simulink model "morus_uav_smc_DOB"  (R2016b)
settings: Solver=FixedStepAuto  StartTime=0.0  StopTime=15  FixedStep=0.001  MaxStep=0.001  RelTol=1e-5  EnableMultiTasking=on
values from neighbouring files (symbols this model uses):
  b_gm_f = F_n / (w_gm_n^2)    (= 0.000456410576724)    [morus_uav_params.m]
  b_gm_m = 0.01    [morus_uav_params.m]
  beta = deg2rad(0)    [morus_uav_params.m]
  cd = 0    [morus_uav_params.m]
  g = 9.81    [morus_uav_params.m]
  Iq = [Iq_xx 0 0; 0 Iq_yy 0; 0 0 Iq_zz]    [morus_uav_params.m]
  Iq_yy = 0.00528250    (= 0.0052825)    [morus_uav_params.m]
  kd_mp = 0.015    [morus_uav_params.m]
  kd_mv = 0.01    [morus_uav_params.m]
  kd_vz = 10    [morus_uav_params.m]
  kd_z = 1    [morus_uav_params.m]
  ki_mp = 0.25    [morus_uav_params.m]
  ki_mv = 06    (= 6)    [morus_uav_params.m]
  ki_vz = 20    [morus_uav_params.m]
  ki_z = 0    [morus_uav_params.m]
  Km = 1    [morus_uav_params.m]
  kp_mp = 25    [morus_uav_params.m]
  kp_mv = 0.6    [morus_uav_params.m]
  kp_vz = 75    [morus_uav_params.m]
  kp_z = 4    [morus_uav_params.m]
  l_rot = 0.265    [morus_uav_params.m]
  lm = 0.17    [morus_uav_params.m]
  m = 0.208    [morus_uav_params.m]
  M = mq + 4 * m    (= 2.915)    [morus_uav_params.m]
  mq = 2.083    [morus_uav_params.m]
  T_obz1 = 5    [morus_uav_params.m]
  T_obz2 = 5    [morus_uav_params.m]
  Tf1 = 0.12    [morus_uav_params.m]
  Tf2 = 0.12    [morus_uav_params.m]
  Tgm = 0.2    [morus_uav_params.m]
  Tr = 12.24268    [morus_uav_params.m]
  w_gm_0 = sqrt(M*g/4/b_gm_f)    [morus_uav_params.m]
  zeta = [1 -1 1 -1]    [morus_uav_params.m]
  zm = 0    [morus_uav_params.m]
libraries: aerolibutil x20, simulink x10, dspmtrx3 x5, aerolibtransform2 x4
(part 1 of 2)
settings Model: Creator=tomislav  LastModifiedBy=martinatomic
settings DataIOCC: LimitDataPoints=on  SaveFormat=Array
settings OptimizationCC: LifeSpan=inf
settings DebuggingCC: SFUnexpectedBacktrackingDiag=warning  SFNoUnconditionalDefaultTransitionDiag=warning  SFExecutionAtInitializationDiag=none
settings HardwareCC: ProdBitPerPointer=32  ProdBitPerSizeT=32  ProdBitPerPtrDiffT=32  ProdLargestAtomicFloat=None  ProdIntDivRoundTo=Undefined  ProdEndianess=Unspecified  ProdWordSize=32  ProdHWDeviceType=32-bit Generic
settings ModelReferenceCC: PropagateSignalLabelsOutOfModel=off
settings GRTTargetCC: TargetLangStandard=C89/C90 (ANSI)  GeneratePreprocessorConditionals=Disable all
settings ConfigComp: CovMetricSettings=dw  CovHtmlReporting=on  CovSaveCumulativeToWorkspaceVar=on  CovSaveSingleToWorkspaceVar=on  CovExternalEMLEnable=off

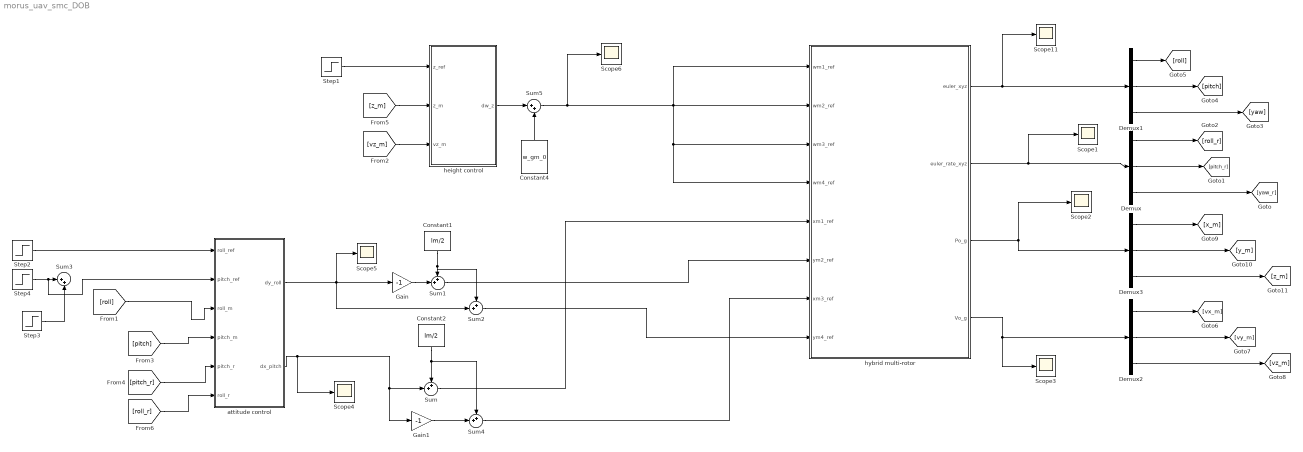
== system morus_uav_smc_DOB ==
  Constant1 : Constant  Value=lm/2
  Constant2 : Constant  Value=lm/2
  Constant4 : Constant  Value=w_gm_0
  Demux{,1..3} (4 alike) : Demux  Outputs=3
  Gain : Gain  Gain=-1
  Gain1 : Gain  Gain=-1
  Scope{1..6,11} (7 alike) : Scope
  Step1 : Step  Time=0  SampleTime=0
  Step2 : Step  Time=5  After=-0.1  SampleTime=0
  Step3 : Step  Time=9  After=0.1  SampleTime=0
  Step4 : Step  Time=5  After=0.1  SampleTime=0
  Sum{,1..2,4} (4 alike) : Sum  Inputs=++|
  Sum3 : Sum  Inputs=|++
  Sum5 : Sum  Inputs=|++
  attitude control : Subsystem
  height control : Subsystem
  hybrid multi-rotor : Subsystem
  wires:
  Sum2/1 -> hybrid multi-rotor/8(ym4_ref)
  hybrid multi-rotor/1(euler_xyz) -> Demux1/1, Scope11/1
  hybrid multi-rotor/2(euler_rate_xyz) -> Demux/1, Scope1/1
  Demux/2 -> [pitch_r]
  Demux1/2 -> [pitch]
  Sum5/1 -> Scope6/1, hybrid multi-rotor/1(wm1_ref), hybrid multi-rotor/4(wm4_ref), hybrid multi-rotor/3(wm3_ref), hybrid multi-rotor/2(wm2_ref)
  height control/1(dw_z) -> Sum5/1
  Constant4/1 -> Sum5/2
  hybrid multi-rotor/4(Vo_g) -> Demux2/1, Scope3/1
  Demux2/2 -> [vy_m]
  Demux2/3 -> [vz_m]
  Demux2/1 -> [vx_m]
  hybrid multi-rotor/3(Po_g) -> Demux3/1, Scope2/1
  Demux3/2 -> [y_m]
  Demux3/3 -> [z_m]
  Demux3/1 -> [x_m]
  [vz_m] -> height control/3(vz_m)
  [z_m] -> height control/2(z_m)
  Step1/1 -> height control/1(z_ref)
  Constant1/1 -> Sum2/1, Sum1/1
  Gain/1 -> Sum1/2
  Constant2/1 -> Sum/1, Sum4/1
  Gain1/1 -> Sum4/2
  Sum/1 -> hybrid multi-rotor/5(xm1_ref)
  Sum1/1 -> hybrid multi-rotor/6(ym2_ref)
  Sum4/1 -> hybrid multi-rotor/7(xm3_ref)
  Step2/1 -> attitude control/1(roll_ref)
  attitude control/2(dx_pitch) -> Sum/2, Gain1/1, Scope4/1
  [pitch] -> attitude control/4(pitch_m)
  [roll] -> attitude control/3(roll_m)
  attitude control/1(dy_roll) -> Scope5/1, Sum2/2, Gain/1
  Demux/1 -> [roll_r]
  Demux/3 -> [yaw_r]
  Demux1/1 -> [roll]
  Demux1/3 -> [yaw]
  [pitch_r] -> attitude control/5(pitch_r)
  [roll_r] -> attitude control/6(roll_r)
  Step4/1 -> attitude control/2(pitch_ref), Sum3/1
  Step3/1 -> Sum3/2

== system morus_uav_smc_DOB/attitude control ==
  roll_ref : Inport
  pitch_ref : Inport  Port=2
  roll_m : Inport  Port=3
  pitch_m : Inport  Port=4
  pitch_r : Inport  Port=5
  roll_r : Inport  Port=6
  pitch control : Subsystem
  roll control : Subsystem
  dy_roll : Outport
  dx_pitch : Outport  Port=2
  wires:
  pitch_ref/1 -> pitch control/1(pitch_ref)
  pitch control/1(dx_pitch) -> dx_pitch/1
  pitch_m/1 -> pitch control/2(pitch_m)
  roll control/1(dy_roll) -> dy_roll/1
  roll_m/1 -> roll control/2(roll_m)
  roll_ref/1 -> roll control/1(roll_ref)
  pitch_r/1 -> pitch control/3(pitch_r)
  roll_r/1 -> roll control/3(roll_r)

== system morus_uav_smc_DOB/height control ==
  z_ref : Inport
  z_m : Inport  Port=2
  vz_m : Inport  Port=3
  Mux : Mux  Inputs=2
  Mux1 : Mux  Inputs=2
  PID Controller : simulink/Continuous/PID Controller  Controller=PID  TimeDomain=Continuous-time  SampleTime=-1  IntegratorMethod=Forward Euler  FilterMethod=Forward Euler  Form=Parallel  UseFilter=on  ControllerParametersSource=internal  P=kp_vz  I=ki_vz  D=kd_vz  N=100  InitialConditionSource=internal  InitialConditionForIntegrator=0  InitialConditionForFilter=0  ExternalReset=none  LimitOutput=on  UpperSaturationLimit=400  LowerSaturationLimit=-400  LinearizeAsGain=on  AntiWindupMode=clamping  Kb=1  TrackingMode=off  Kt=1  PParamMin=[]  PParamMax=[]  IParamMin=[]  IParamMax=[]  DParamMin=[]  DParamMax=[]  NParamMin=[]  NParamMax=[]  KbParamMin=[]  KbParamMax=[]  KtParamMin=[]  KtParamMax=[]  POutMin=[]  POutMax=[]  IOutMin=[]  IOutMax=[]  DOutMin=[]  DOutMax=[]  NOutMin=[]  NOutMax=[]  KbOutMin=[]  KbOutMax=[]  KtOutMin=[]  KtOutMax=[]  IntegratorOutMin=[]  IntegratorOutMax=[]  FilterOutMin=[]  FilterOutMax=[]  SumOutMin=[]  SumOutMax=[]  SumI1OutMin=[]  SumI1OutMax=[]  SumI2OutMin=[]  SumI2OutMax=[]  SumI3OutMin=[]  SumI3OutMax=[]  SumDOutMin=[]  SumDOutMax=[]  SaturationOutMin=[]  SaturationOutMax=[]  IntegratorContinuousStateAttributes=''  IntegratorStateMustResolveToSignalObject=off  IntegratorRTWStateStorageClass=Auto  FilterContinuousStateAttributes=''  FilterStateMustResolveToSignalObject=off  FilterRTWStateStorageClass=Auto  DifferentiatorICPrevScaledInput=0  DifferentiatorOutMin=[]  DifferentiatorOutMax=[]
  PID Controller1 : simulink/Continuous/PID Controller  Controller=PID  TimeDomain=Continuous-time  SampleTime=-1  IntegratorMethod=Forward Euler  FilterMethod=Forward Euler  Form=Parallel  UseFilter=on  ControllerParametersSource=internal  P=kp_z  I=ki_z  D=kd_z  N=100  InitialConditionSource=internal  InitialConditionForIntegrator=0  InitialConditionForFilter=0  ExternalReset=none  LimitOutput=on  UpperSaturationLimit=5  LowerSaturationLimit=-5  LinearizeAsGain=on  AntiWindupMode=clamping  Kb=1  TrackingMode=off  Kt=1  PParamMin=[]  PParamMax=[]  IParamMin=[]  IParamMax=[]  DParamMin=[]  DParamMax=[]  NParamMin=[]  NParamMax=[]  KbParamMin=[]  KbParamMax=[]  KtParamMin=[]  KtParamMax=[]  POutMin=[]  POutMax=[]  IOutMin=[]  IOutMax=[]  DOutMin=[]  DOutMax=[]  NOutMin=[]  NOutMax=[]  KbOutMin=[]  KbOutMax=[]  KtOutMin=[]  KtOutMax=[]  IntegratorOutMin=[]  IntegratorOutMax=[]  FilterOutMin=[]  FilterOutMax=[]  SumOutMin=[]  SumOutMax=[]  SumI1OutMin=[]  SumI1OutMax=[]  SumI2OutMin=[]  SumI2OutMax=[]  SumI3OutMin=[]  SumI3OutMax=[]  SumDOutMin=[]  SumDOutMax=[]  SaturationOutMin=[]  SaturationOutMax=[]  IntegratorContinuousStateAttributes=''  IntegratorStateMustResolveToSignalObject=off  IntegratorRTWStateStorageClass=Auto  FilterContinuousStateAttributes=''  FilterStateMustResolveToSignalObject=off  FilterRTWStateStorageClass=Auto  DifferentiatorICPrevScaledInput=0  DifferentiatorOutMin=[]  DifferentiatorOutMax=[]
  Scope1 : Scope
  Scope4 : Scope
  Scope6 : Scope
  Sum : Sum  Inputs=|+-
  Sum1 : Sum  Inputs=|+-
  dw_z : Outport
  wires:
  z_m/1 -> Sum1/2, Mux1/2
  Mux1/1 -> Scope6/1
  z_ref/1 -> Sum1/1, Mux1/1
  Sum/1 -> PID Controller/1
  Sum1/1 -> PID Controller1/1
  Mux/1 -> Scope4/1
  vz_m/1 -> Sum/2, Mux/2
  PID Controller1/1 -> Sum/1, Mux/1
  PID Controller/1 -> Scope1/1, dw_z/1

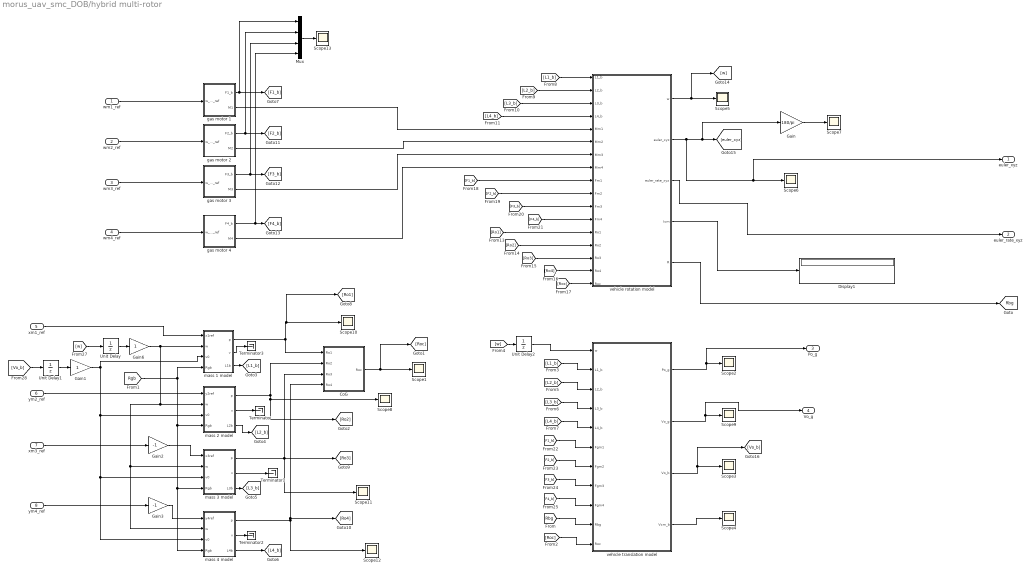
== system morus_uav_smc_DOB/hybrid multi-rotor ==
  wm1_ref : Inport
  wm2_ref : Inport  Port=2
  wm3_ref : Inport  Port=3
  wm4_ref : Inport  Port=4
  xm1_ref : Inport  Port=5
  ym2_ref : Inport  Port=6
  xm3_ref : Inport  Port=7
  ym4_ref : Inport  Port=8
  CoG : Subsystem
  Display1 : Display
  Gain : Gain  Gain=180/pi
  Gain1 : Gain
  Gain2 : Gain  Gain=-1
  Gain3 : Gain  Gain=-1
  Gain6 : Gain
  Mux : Mux
  Scope{1..13} (13 alike) : Scope
  Terminator{,1..3} (4 alike) : Terminator
  Unit Delay : UnitDelay  SampleTime=-1
  Unit Delay1 : UnitDelay  SampleTime=-1
  Unit Delay2 : UnitDelay  SampleTime=-1
  gas motor 1 : Subsystem
  gas motor 2 : Subsystem
  gas motor 3 : Subsystem
  gas motor 4 : Subsystem
  mass 1 model : Subsystem
  mass 2 model : Subsystem
  mass 3 model : Subsystem
  mass 4 model : Subsystem
  vehicle rotation model : Subsystem
  vehicle translation model : Subsystem
  euler_xyz : Outport
  euler_rate_xyz : Outport  Port=2
  Po_g : Outport  Port=3
  Vo_g : Outport  Port=4
  tag scope: Rbg=global
  wires:
  vehicle rotation model/3(euler_rate_xyz) -> euler_rate_xyz/1
  [Rbg] -> vehicle translation model/10(Rbg)
  mass 2 model/1(p) -> Scope8/1, [Ro2], CoG/2(Ro2)
  mass 3 model/1(p) -> CoG/3(Ro3), Scope11/1, [Ro3]
  mass 4 model/1(p) -> [Ro4], CoG/4(Ro4), Scope12/1
  [Roc] -> vehicle translation model/11(Roc)
  vehicle translation model/2(Vo_g) -> Vo_g/1, Scope9/1
  [Roc] -> vehicle rotation model/17(Roc)
  Gain2/1 -> mass 3 model/1(x3ref)
  [L1_b] -> vehicle rotation model/1(L1_b)
  mass 3 model/3(L3b) -> [L3_b]
  [L4_b] -> vehicle translation model/5(L4_b)
  [L2_b] -> vehicle translation model/3(L2_b)
  [Ro3] -> vehicle rotation model/15(Ro3)
  vehicle translation model/1(Po_g) -> Po_g/1, Scope2/1
  vehicle translation model/3(Vo_b) -> [Vo_b], Scope3/1
  mass 2 model/3(L2b) -> [L2_b]
  vehicle translation model/4(Vcm_b) -> Scope4/1
  xm1_ref/1 -> mass 1 model/1(x1ref)
  [Ro1] -> vehicle rotation model/13(Ro1)
  Gain3/1 -> mass 4 model/1(y4ref)
  [L3_b] -> vehicle rotation model/3(L3_b)
  [L3_b] -> vehicle translation model/4(L3_b)
  mass 1 model/3(L1b) -> [L1_b]
  [L2_b] -> vehicle rotation model/2(L2_b)
  [Ro4] -> vehicle rotation model/16(Ro4)
  [L1_b] -> vehicle translation model/2(L1_b)
  ym4_ref/1 -> Gain3/1
  [Ro2] -> vehicle rotation model/14(Ro2)
  vehicle rotation model/1(w) -> [w], Scope5/1
  vehicle rotation model/4(Icm) -> Display1/1
  ym2_ref/1 -> mass 2 model/1(y2ref)
  mass 4 model/3(L4b) -> [L4_b]
  xm3_ref/1 -> Gain2/1
  [F4_b] -> vehicle rotation model/12(Fm4)
  gas motor 2/1(F2_b) -> Mux/2, [F2_b]
  wm4_ref/1 -> gas motor 4/1(w_gm4_ref)
  vehicle rotation model/2(euler_xyz) -> euler_xyz/1, Scope6/1, [euler_xyz], Gain/1
  CoG/1(Roc) -> [Roc], Scope1/1
  [F2_b] -> vehicle rotation model/10(Fm2)
  wm1_ref/1 -> gas motor 1/1(w_gm1_ref)
  [F1_b] -> vehicle rotation model/9(Fm1)
  gas motor 4/1(F4_b) -> Mux/4, [F4_b]
  gas motor 1/1(F1_b) -> Mux/1, [F1_b]
  gas motor 3/2(M3) -> vehicle rotation model/7(Mm3)
  [F3_b] -> vehicle rotation model/11(Fm3)
  gas motor 1/2(M1) -> vehicle rotation model/5(Mm1)
  [F2_b] -> vehicle translation model/7(Fgm2)
  [F1_b] -> vehicle translation model/6(Fgm1)
  gas motor 2/2(M2) -> vehicle rotation model/6(Mm2)
  gas motor 3/1(F3_b) -> Mux/3, [F3_b]
  [Vo_b] -> Unit Delay1/1
  [F3_b] -> vehicle translation model/8(Fgm3)
  [L4_b] -> vehicle rotation model/4(L4_b)
  [F4_b] -> vehicle translation model/9(Fgm4)
  gas motor 4/2(M4) -> vehicle rotation model/8(Mm4)
  wm2_ref/1 -> gas motor 2/1(w_gm2_ref)
  wm3_ref/1 -> gas motor 3/1(w_gm3_ref)
  mass 2 model/2(v) -> Terminator/1
  mass 1 model/2(v) -> Terminator3/1
  mass 4 model/2(v) -> Terminator2/1
  Gain/1 -> Scope7/1
  mass 1 model/1(p) -> CoG/1(Ro1), [Ro1], Scope10/1
  [w] -> Unit Delay/1
  [w] -> Unit Delay2/1
  Unit Delay2/1 -> vehicle translation model/1(w)
  [Rgb] -> mass 1 model/4(Rgb), mass 2 model/4(Rgb), mass 3 model/4(Rgb), mass 4 model/4(Rgb)
  Unit Delay/1 -> Gain6/1
  Unit Delay1/1 -> Gain1/1
  Gain6/1 -> mass 1 model/2(w), mass 4 model/2(w), mass 3 model/2(w), mass 2 model/2(w)
  Gain1/1 -> mass 1 model/3(v0), mass 4 model/3(v0), mass 3 model/3(v0), mass 2 model/3(v0)
  Mux/1 -> Scope13/1
  mass 3 model/2(v) -> Terminator1/1
  vehicle rotation model/5(R) -> [Rbg]

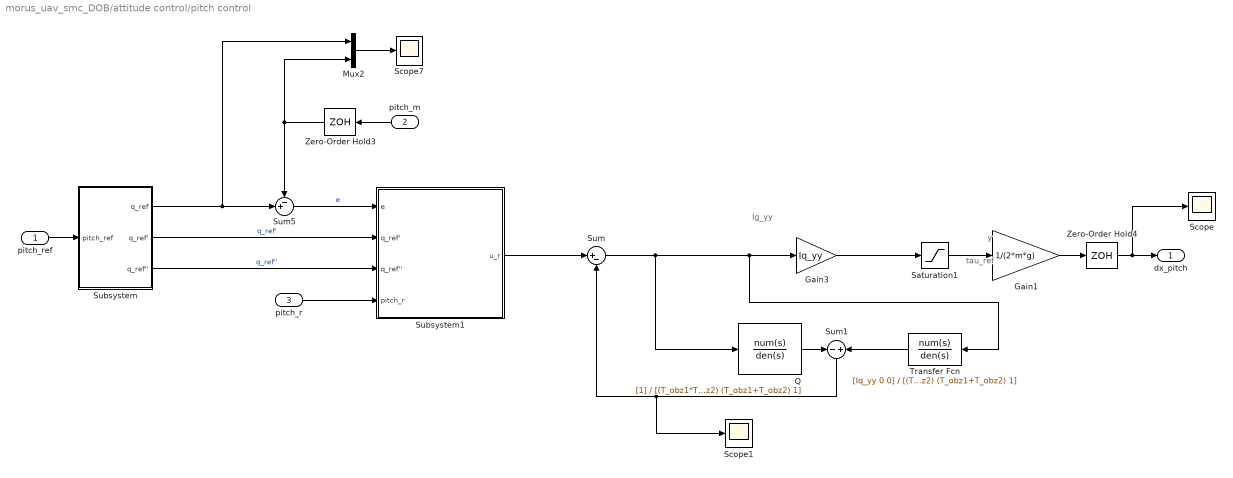
== system morus_uav_smc_DOB/attitude control/pitch control ==
  note: y
  note: Ig_yy
  note: tau_ref
  pitch_ref : Inport
  pitch_m : Inport  Port=2
  pitch_r : Inport  Port=3
  Gain1 : Gain  Gain=1/(2*m*g)
  Gain3 : Gain  Gain=Iq_yy
  Mux2 : Mux  Inputs=2
  Q : TransferFcn  Denominator=[(T_obz1*T_obz2) (T_obz1+T_obz2) 1]
  Saturation1 : Saturate  UpperLimit=lm/2  LowerLimit=-lm/2
  Scope : Scope
  Scope1 : Scope
  Scope7 : Scope
  Subsystem : Subsystem
  Subsystem1 : Subsystem
  Sum : Sum  Inputs=|+-
  Sum1 : Sum  Inputs=-|+
  Sum5 : Sum  Inputs=-+|
  Transfer Fcn : TransferFcn  Numerator=[Iq_yy 0 0]  Denominator=[(T_obz1*T_obz2) (T_obz1+T_obz2) 1]
  Zero-Order Hold3 : ZeroOrderHold  SampleTime=0.001
  Zero-Order Hold4 : ZeroOrderHold  SampleTime=-1
  dx_pitch : Outport
  wires:
  Mux2/1 -> Scope7/1
  pitch_m/1 -> Zero-Order Hold3/1
  Saturation1/1 -> Gain1/1
  Zero-Order Hold4/1 -> Scope/1, dx_pitch/1
  pitch_ref/1 -> Subsystem/1(pitch_ref)
  Subsystem/1(q_ref) -> Sum5/2, Mux2/1
  Gain3/1 -> Saturation1/1
  Zero-Order Hold3/1 -> Sum5/1, Mux2/2
  Sum5/1 -> Subsystem1/1(e)  "e"
  Subsystem/2(q_ref') -> Subsystem1/2(q_ref')  "q_ref'"
  Subsystem/3(q_ref'') -> Subsystem1/3(q_ref'')  "q_ref''"
  pitch_r/1 -> Subsystem1/4(pitch_r)
  Subsystem1/1(u_r) -> Sum/1
  Sum/1 -> Q/1, Transfer Fcn/1, Gain3/1
  Q/1 -> Sum1/1
  Transfer Fcn/1 -> Sum1/2
  Sum1/1 -> Scope1/1, Sum/2
  Gain1/1 -> Zero-Order Hold4/1

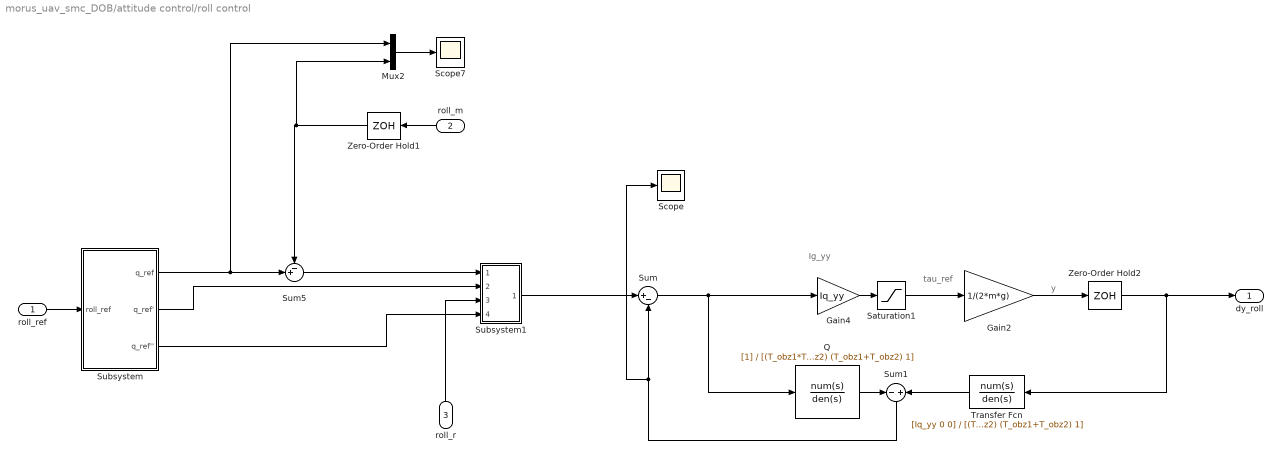
== system morus_uav_smc_DOB/attitude control/roll control ==
  note: y
  note: Ig_yy
  note: tau_ref
  roll_ref : Inport
  roll_m : Inport  Port=2
  roll_r : Inport  Port=3
  Gain2 : Gain  Gain=1/(2*m*g)
  Gain4 : Gain  Gain=Iq_yy
  Mux2 : Mux  Inputs=2
  Q : TransferFcn  Denominator=[(T_obz1*T_obz2) (T_obz1+T_obz2) 1]
  Saturation1 : Saturate  UpperLimit=lm/2  LowerLimit=-lm/2
  Scope : Scope
  Scope7 : Scope
  Subsystem : Subsystem
  Subsystem1 : Subsystem
  Sum : Sum  Inputs=|+-
  Sum1 : Sum  Inputs=-|+
  Sum5 : Sum  Inputs=-+|
  Transfer Fcn : TransferFcn  Numerator=[Iq_yy 0 0]  Denominator=[(T_obz1*T_obz2) (T_obz1+T_obz2) 1]
  Zero-Order Hold1 : ZeroOrderHold  SampleTime=0.001
  Zero-Order Hold2 : ZeroOrderHold  SampleTime=-1
  dy_roll : Outport
  wires:
  Mux2/1 -> Scope7/1
  roll_m/1 -> Zero-Order Hold1/1
  roll_ref/1 -> Subsystem/1(roll_ref)
  Subsystem/1(q_ref) -> Sum5/2, Mux2/1
  Zero-Order Hold1/1 -> Mux2/2, Sum5/1
  Sum5/1 -> Subsystem1/1(In1)
  Subsystem/2(q_ref') -> Subsystem1/2(In2)
  roll_r/1 -> Subsystem1/3(roll_r)
  Subsystem/3(q_ref'') -> Subsystem1/4(In4)
  Saturation1/1 -> Gain2/1
  Gain4/1 -> Saturation1/1
  Subsystem1/1(Out1) -> Sum/1
  Sum/1 -> Q/1, Gain4/1
  Q/1 -> Sum1/1
  Transfer Fcn/1 -> Sum1/2
  Gain2/1 -> Zero-Order Hold2/1
  Sum1/1 -> Scope/1, Sum/2
  Zero-Order Hold2/1 -> dy_roll/1, Transfer Fcn/1

== system morus_uav_smc_DOB/hybrid multi-rotor/CoG ==
  note: Roc
  Ro1 : Inport
  Ro2 : Inport  Port=2
  Ro3 : Inport  Port=3
  Ro4 : Inport  Port=4
  Gain : Gain  Gain=m/M
  Sum3 : Sum  Inputs=++++
  Roc : Outport
  wires:
  Sum3/1 -> Gain/1
  Gain/1 -> Roc/1
  Ro3/1 -> Sum3/3
  Ro2/1 -> Sum3/2
  Ro4/1 -> Sum3/4
  Ro1/1 -> Sum3/1

== system morus_uav_smc_DOB/hybrid multi-rotor/gas motor 1 ==
  note: w_gm
  w_gm1_ref : Inport
  Constant1 : Constant  Value=0
  Constant6 : Constant  Value=0
  Gain : Gain  Gain=b_gm_f
  Gain1 : Gain  Gain=b_gm_m
  Gain2 : Gain  Gain=1/Tgm
  Integrator : Integrator  InitialCondition=w_gm_0
  Math Function : Math  Operator=square  SaturateOnIntegerOverflow=on
  Mux1 : Mux  Inputs=3
  Mux4 : Mux  Inputs=3
  Scope5 : Scope
  Sum : Sum  Inputs=|+-
  cw : Gain  Gain=zeta(1)
  F1_b : Outport
  M1 : Outport  Port=2
  wires:
  w_gm1_ref/1 -> Sum/1
  Gain/1 -> Gain1/1, Mux4/3
  Math Function/1 -> Gain/1
  Constant6/1 -> Mux4/2, Mux4/1
  Mux4/1 -> F1_b/1
  Constant1/1 -> Mux1/2, Mux1/1
  cw/1 -> Mux1/3
  Gain1/1 -> cw/1
  Mux1/1 -> M1/1
  Sum/1 -> Gain2/1
  Gain2/1 -> Integrator/1
  Integrator/1 -> Sum/2, Math Function/1, Scope5/1

== system morus_uav_smc_DOB/hybrid multi-rotor/gas motor 2 ==
  note: w_gm
  w_gm2_ref : Inport
  Constant1 : Constant  Value=0
  Constant6 : Constant  Value=0
  Gain : Gain  Gain=b_gm_f
  Gain1 : Gain  Gain=b_gm_m
  Gain2 : Gain  Gain=1/Tgm
  Integrator : Integrator  InitialCondition=w_gm_0
  Math Function : Math  Operator=square  SaturateOnIntegerOverflow=on
  Mux1 : Mux  Inputs=3
  Mux4 : Mux  Inputs=3
  Scope1 : Scope
  Scope11 : Scope
  Sum : Sum  Inputs=|+-
  cw : Gain  Gain=zeta(2)
  F2_b : Outport
  M2 : Outport  Port=2
  wires:
  Mux1/1 -> M2/1
  Gain1/1 -> cw/1
  cw/1 -> Mux1/3
  Constant1/1 -> Mux1/1, Mux1/2
  Mux4/1 -> F2_b/1
  Constant6/1 -> Mux4/1, Mux4/2
  Math Function/1 -> Gain/1
  Gain/1 -> Scope11/1, Mux4/3, Gain1/1
  w_gm2_ref/1 -> Sum/1
  Sum/1 -> Gain2/1
  Gain2/1 -> Integrator/1
  Integrator/1 -> Scope1/1, Math Function/1, Sum/2

== system morus_uav_smc_DOB/hybrid multi-rotor/gas motor 3 ==
  note: w_gm
  w_gm3_ref : Inport
  Constant1 : Constant  Value=0
  Constant6 : Constant  Value=0
  Gain : Gain  Gain=b_gm_f
  Gain1 : Gain  Gain=b_gm_m
  Gain2 : Gain  Gain=1/Tgm
  Integrator : Integrator  InitialCondition=w_gm_0
  Math Function : Math  Operator=square  SaturateOnIntegerOverflow=on
  Mux1 : Mux  Inputs=3
  Mux4 : Mux  Inputs=3
  Sum : Sum  Inputs=|+-
  cw : Gain  Gain=zeta(3)
  F3_b : Outport
  M3 : Outport  Port=2
  wires:
  Gain/1 -> Gain1/1, Mux4/3
  Math Function/1 -> Gain/1
  Constant6/1 -> Mux4/2, Mux4/1
  Mux4/1 -> F3_b/1
  Constant1/1 -> Mux1/2, Mux1/1
  cw/1 -> Mux1/3
  Gain1/1 -> cw/1
  Mux1/1 -> M3/1
  w_gm3_ref/1 -> Sum/1
  Sum/1 -> Gain2/1
  Gain2/1 -> Integrator/1
  Integrator/1 -> Math Function/1, Sum/2

== system morus_uav_smc_DOB/hybrid multi-rotor/gas motor 4 ==
  note: w_gm
  w_gm4_ref : Inport
  Constant1 : Constant  Value=0
  Constant6 : Constant  Value=0
  Gain : Gain  Gain=b_gm_f
  Gain1 : Gain  Gain=b_gm_m
  Gain2 : Gain  Gain=1/Tgm
  Integrator : Integrator  InitialCondition=w_gm_0
  Math Function : Math  Operator=square  SaturateOnIntegerOverflow=on
  Mux1 : Mux  Inputs=3
  Mux4 : Mux  Inputs=3
  Sum : Sum  Inputs=|+-
  cw : Gain  Gain=zeta(4)
  F4_b : Outport
  M4 : Outport  Port=2
  wires:
  Mux1/1 -> M4/1
  Gain1/1 -> cw/1
  cw/1 -> Mux1/3
  Constant1/1 -> Mux1/1, Mux1/2
  Mux4/1 -> F4_b/1
  Constant6/1 -> Mux4/1, Mux4/2
  Math Function/1 -> Gain/1
  Gain/1 -> Mux4/3, Gain1/1
  w_gm4_ref/1 -> Sum/1
  Sum/1 -> Gain2/1
  Gain2/1 -> Integrator/1
  Integrator/1 -> Math Function/1, Sum/2

== system morus_uav_smc_DOB/hybrid multi-rotor/mass 1 model ==
  note: PT2S modelirati
  x1ref : Inport
  w : Inport  Port=2
  v0 : Inport  Port=3
  Rgb : Inport  Port=4
  PID Controller : simulink/Continuous/PID Controller  Controller=PID  TimeDomain=Continuous-time  SampleTime=-1  IntegratorMethod=Forward Euler  FilterMethod=Forward Euler  Form=Parallel  UseFilter=on  ControllerParametersSource=internal  P=kp_mv  I=ki_mv  D=kd_mv  N=100  InitialConditionSource=internal  InitialConditionForIntegrator=0  InitialConditionForFilter=0  ExternalReset=none  LimitOutput=off  UpperSaturationLimit=12  LowerSaturationLimit=-12  LinearizeAsGain=on  AntiWindupMode=clamping  Kb=1  TrackingMode=off  Kt=1  PParamMin=[]  PParamMax=[]  IParamMin=[]  IParamMax=[]  DParamMin=[]  DParamMax=[]  NParamMin=[]  NParamMax=[]  KbParamMin=[]  KbParamMax=[]  KtParamMin=[]  KtParamMax=[]  POutMin=[]  POutMax=[]  IOutMin=[]  IOutMax=[]  DOutMin=[]  DOutMax=[]  NOutMin=[]  NOutMax=[]  KbOutMin=[]  KbOutMax=[]  KtOutMin=[]  KtOutMax=[]  IntegratorOutMin=[]  IntegratorOutMax=[]  FilterOutMin=[]  FilterOutMax=[]  SumOutMin=[]  SumOutMax=[]  SumI1OutMin=[]  SumI1OutMax=[]  SumI2OutMin=[]  SumI2OutMax=[]  SumI3OutMin=[]  SumI3OutMax=[]  SumDOutMin=[]  SumDOutMax=[]  SaturationOutMin=[]  SaturationOutMax=[]  IntegratorContinuousStateAttributes=''  IntegratorStateMustResolveToSignalObject=off  IntegratorRTWStateStorageClass=Auto  FilterContinuousStateAttributes=''  FilterStateMustResolveToSignalObject=off  FilterRTWStateStorageClass=Auto  DifferentiatorICPrevScaledInput=0  DifferentiatorOutMin=[]  DifferentiatorOutMax=[]
  PID Controller1 : simulink/Continuous/PID Controller  Controller=PID  TimeDomain=Continuous-time  SampleTime=-1  IntegratorMethod=Forward Euler  FilterMethod=Forward Euler  Form=Parallel  UseFilter=on  ControllerParametersSource=internal  P=kp_mp  I=ki_mp  D=kd_mp  N=100  InitialConditionSource=internal  InitialConditionForIntegrator=0  InitialConditionForFilter=0  ExternalReset=none  LimitOutput=off  UpperSaturationLimit=12  LowerSaturationLimit=-12  LinearizeAsGain=on  AntiWindupMode=clamping  Kb=1  TrackingMode=off  Kt=1  PParamMin=[]  PParamMax=[]  IParamMin=[]  IParamMax=[]  DParamMin=[]  DParamMax=[]  NParamMin=[]  NParamMax=[]  KbParamMin=[]  KbParamMax=[]  KtParamMin=[]  KtParamMax=[]  POutMin=[]  POutMax=[]  IOutMin=[]  IOutMax=[]  DOutMin=[]  DOutMax=[]  NOutMin=[]  NOutMax=[]  KbOutMin=[]  KbOutMax=[]  KtOutMin=[]  KtOutMax=[]  IntegratorOutMin=[]  IntegratorOutMax=[]  FilterOutMin=[]  FilterOutMax=[]  SumOutMin=[]  SumOutMax=[]  SumI1OutMin=[]  SumI1OutMax=[]  SumI2OutMin=[]  SumI2OutMax=[]  SumI3OutMin=[]  SumI3OutMax=[]  SumDOutMin=[]  SumDOutMax=[]  SaturationOutMin=[]  SaturationOutMax=[]  IntegratorContinuousStateAttributes=''  IntegratorStateMustResolveToSignalObject=off  IntegratorRTWStateStorageClass=Auto  FilterContinuousStateAttributes=''  FilterStateMustResolveToSignalObject=off  FilterRTWStateStorageClass=Auto  DifferentiatorICPrevScaledInput=0  DifferentiatorOutMin=[]  DifferentiatorOutMax=[]
  Scope{2..5} (4 alike) : Scope
  Sum : Sum  Inputs=|+-
  Sum1 : Sum  Inputs=|+-  OutDataTypeStr=Inherit: Same as first input
  mass dynamics through L : Subsystem
  p : Outport
  v : Outport  Port=2
  L1b : Outport  Port=3
  wires:
  PID Controller/1 -> mass dynamics through L/1(U), Scope3/1
  Sum/1 -> PID Controller/1
  Sum1/1 -> PID Controller1/1
  PID Controller1/1 -> Sum/1, Scope2/1
  w/1 -> mass dynamics through L/2(w)
  v0/1 -> mass dynamics through L/3(v0)
  Rgb/1 -> mass dynamics through L/4(Rgb)
  mass dynamics through L/5(vx_a) -> v/1, Sum/2
  mass dynamics through L/4(x_a) -> Sum1/2
  mass dynamics through L/1(p_b) -> Scope4/1, p/1
  mass dynamics through L/3(L) -> Scope5/1
  mass dynamics through L/6(L1b) -> L1b/1
  x1ref/1 -> Sum1/1

== system morus_uav_smc_DOB/hybrid multi-rotor/mass 2 model ==
  y2ref : Inport
  w : Inport  Port=2
  v0 : Inport  Port=3
  Rgb : Inport  Port=4
  PID Controller : simulink/Continuous/PID Controller  Controller=PID  TimeDomain=Continuous-time  SampleTime=-1  IntegratorMethod=Forward Euler  FilterMethod=Forward Euler  Form=Parallel  UseFilter=on  ControllerParametersSource=internal  P=kp_mv  I=ki_mv  D=kd_mv  N=100  InitialConditionSource=internal  InitialConditionForIntegrator=0  InitialConditionForFilter=0  ExternalReset=none  LimitOutput=off  UpperSaturationLimit=12  LowerSaturationLimit=-12  LinearizeAsGain=on  AntiWindupMode=clamping  Kb=1  TrackingMode=off  Kt=1  PParamMin=[]  PParamMax=[]  IParamMin=[]  IParamMax=[]  DParamMin=[]  DParamMax=[]  NParamMin=[]  NParamMax=[]  KbParamMin=[]  KbParamMax=[]  KtParamMin=[]  KtParamMax=[]  POutMin=[]  POutMax=[]  IOutMin=[]  IOutMax=[]  DOutMin=[]  DOutMax=[]  NOutMin=[]  NOutMax=[]  KbOutMin=[]  KbOutMax=[]  KtOutMin=[]  KtOutMax=[]  IntegratorOutMin=[]  IntegratorOutMax=[]  FilterOutMin=[]  FilterOutMax=[]  SumOutMin=[]  SumOutMax=[]  SumI1OutMin=[]  SumI1OutMax=[]  SumI2OutMin=[]  SumI2OutMax=[]  SumI3OutMin=[]  SumI3OutMax=[]  SumDOutMin=[]  SumDOutMax=[]  SaturationOutMin=[]  SaturationOutMax=[]  IntegratorContinuousStateAttributes=''  IntegratorStateMustResolveToSignalObject=off  IntegratorRTWStateStorageClass=Auto  FilterContinuousStateAttributes=''  FilterStateMustResolveToSignalObject=off  FilterRTWStateStorageClass=Auto  DifferentiatorICPrevScaledInput=0  DifferentiatorOutMin=[]  DifferentiatorOutMax=[]
  PID Controller1 : simulink/Continuous/PID Controller  Controller=PID  TimeDomain=Continuous-time  SampleTime=-1  IntegratorMethod=Forward Euler  FilterMethod=Forward Euler  Form=Parallel  UseFilter=on  ControllerParametersSource=internal  P=kp_mp  I=ki_mp  D=kd_mp  N=100  InitialConditionSource=internal  InitialConditionForIntegrator=0  InitialConditionForFilter=0  ExternalReset=none  LimitOutput=off  UpperSaturationLimit=12  LowerSaturationLimit=-12  LinearizeAsGain=on  AntiWindupMode=clamping  Kb=1  TrackingMode=off  Kt=1  PParamMin=[]  PParamMax=[]  IParamMin=[]  IParamMax=[]  DParamMin=[]  DParamMax=[]  NParamMin=[]  NParamMax=[]  KbParamMin=[]  KbParamMax=[]  KtParamMin=[]  KtParamMax=[]  POutMin=[]  POutMax=[]  IOutMin=[]  IOutMax=[]  DOutMin=[]  DOutMax=[]  NOutMin=[]  NOutMax=[]  KbOutMin=[]  KbOutMax=[]  KtOutMin=[]  KtOutMax=[]  IntegratorOutMin=[]  IntegratorOutMax=[]  FilterOutMin=[]  FilterOutMax=[]  SumOutMin=[]  SumOutMax=[]  SumI1OutMin=[]  SumI1OutMax=[]  SumI2OutMin=[]  SumI2OutMax=[]  SumI3OutMin=[]  SumI3OutMax=[]  SumDOutMin=[]  SumDOutMax=[]  SaturationOutMin=[]  SaturationOutMax=[]  IntegratorContinuousStateAttributes=''  IntegratorStateMustResolveToSignalObject=off  IntegratorRTWStateStorageClass=Auto  FilterContinuousStateAttributes=''  FilterStateMustResolveToSignalObject=off  FilterRTWStateStorageClass=Auto  DifferentiatorICPrevScaledInput=0  DifferentiatorOutMin=[]  DifferentiatorOutMax=[]
  Scope{1..5} (5 alike) : Scope
  Sum : Sum  Inputs=|+-
  Sum1 : Sum  Inputs=|+-
  mass dynamics through L : Subsystem
  p : Outport
  v : Outport  Port=2
  L2b : Outport  Port=3
  wires:
  Sum/1 -> PID Controller/1
  Sum1/1 -> PID Controller1/1
  PID Controller1/1 -> Sum/1, Scope2/1
  w/1 -> mass dynamics through L/2(w)
  v0/1 -> mass dynamics through L/3(v0)
  Rgb/1 -> mass dynamics through L/4(Rgb)
  mass dynamics through L/5(vy_a) -> v/1, Sum/2
  mass dynamics through L/4(y_a) -> Sum1/2
  mass dynamics through L/1(p_b) -> Scope4/1, p/1
  PID Controller/1 -> mass dynamics through L/1(U), Scope3/1
  mass dynamics through L/3(dL) -> Scope5/1
  mass dynamics through L/6(L2b) -> L2b/1
  y2ref/1 -> Sum1/1

== system morus_uav_smc_DOB/hybrid multi-rotor/mass 3 model ==
  x3ref : Inport
  w : Inport  Port=2
  v0 : Inport  Port=3
  Rgb : Inport  Port=4
  PID Controller : simulink/Continuous/PID Controller  Controller=PID  TimeDomain=Continuous-time  SampleTime=-1  IntegratorMethod=Forward Euler  FilterMethod=Forward Euler  Form=Parallel  UseFilter=on  ControllerParametersSource=internal  P=kp_mv  I=ki_mv  D=kd_mv  N=100  InitialConditionSource=internal  InitialConditionForIntegrator=0  InitialConditionForFilter=0  ExternalReset=none  LimitOutput=off  UpperSaturationLimit=12  LowerSaturationLimit=-12  LinearizeAsGain=on  AntiWindupMode=clamping  Kb=1  TrackingMode=off  Kt=1  PParamMin=[]  PParamMax=[]  IParamMin=[]  IParamMax=[]  DParamMin=[]  DParamMax=[]  NParamMin=[]  NParamMax=[]  KbParamMin=[]  KbParamMax=[]  KtParamMin=[]  KtParamMax=[]  POutMin=[]  POutMax=[]  IOutMin=[]  IOutMax=[]  DOutMin=[]  DOutMax=[]  NOutMin=[]  NOutMax=[]  KbOutMin=[]  KbOutMax=[]  KtOutMin=[]  KtOutMax=[]  IntegratorOutMin=[]  IntegratorOutMax=[]  FilterOutMin=[]  FilterOutMax=[]  SumOutMin=[]  SumOutMax=[]  SumI1OutMin=[]  SumI1OutMax=[]  SumI2OutMin=[]  SumI2OutMax=[]  SumI3OutMin=[]  SumI3OutMax=[]  SumDOutMin=[]  SumDOutMax=[]  SaturationOutMin=[]  SaturationOutMax=[]  IntegratorContinuousStateAttributes=''  IntegratorStateMustResolveToSignalObject=off  IntegratorRTWStateStorageClass=Auto  FilterContinuousStateAttributes=''  FilterStateMustResolveToSignalObject=off  FilterRTWStateStorageClass=Auto  DifferentiatorICPrevScaledInput=0  DifferentiatorOutMin=[]  DifferentiatorOutMax=[]
  PID Controller1 : simulink/Continuous/PID Controller  Controller=PID  TimeDomain=Continuous-time  SampleTime=-1  IntegratorMethod=Forward Euler  FilterMethod=Forward Euler  Form=Parallel  UseFilter=on  ControllerParametersSource=internal  P=kp_mp  I=ki_mp  D=kd_mp  N=100  InitialConditionSource=internal  InitialConditionForIntegrator=0  InitialConditionForFilter=0  ExternalReset=none  LimitOutput=off  UpperSaturationLimit=12  LowerSaturationLimit=-12  LinearizeAsGain=on  AntiWindupMode=clamping  Kb=1  TrackingMode=off  Kt=1  PParamMin=[]  PParamMax=[]  IParamMin=[]  IParamMax=[]  DParamMin=[]  DParamMax=[]  NParamMin=[]  NParamMax=[]  KbParamMin=[]  KbParamMax=[]  KtParamMin=[]  KtParamMax=[]  POutMin=[]  POutMax=[]  IOutMin=[]  IOutMax=[]  DOutMin=[]  DOutMax=[]  NOutMin=[]  NOutMax=[]  KbOutMin=[]  KbOutMax=[]  KtOutMin=[]  KtOutMax=[]  IntegratorOutMin=[]  IntegratorOutMax=[]  FilterOutMin=[]  FilterOutMax=[]  SumOutMin=[]  SumOutMax=[]  SumI1OutMin=[]  SumI1OutMax=[]  SumI2OutMin=[]  SumI2OutMax=[]  SumI3OutMin=[]  SumI3OutMax=[]  SumDOutMin=[]  SumDOutMax=[]  SaturationOutMin=[]  SaturationOutMax=[]  IntegratorContinuousStateAttributes=''  IntegratorStateMustResolveToSignalObject=off  IntegratorRTWStateStorageClass=Auto  FilterContinuousStateAttributes=''  FilterStateMustResolveToSignalObject=off  FilterRTWStateStorageClass=Auto  DifferentiatorICPrevScaledInput=0  DifferentiatorOutMin=[]  DifferentiatorOutMax=[]
  Scope{1..5} (5 alike) : Scope
  Sum : Sum  Inputs=|+-
  Sum1 : Sum  Inputs=|+-
  mass dynamics through L1 : Subsystem
  p : Outport
  v : Outport  Port=2
  L3b : Outport  Port=3
  wires:
  Sum/1 -> PID Controller/1
  Sum1/1 -> PID Controller1/1
  PID Controller1/1 -> Sum/1, Scope2/1
  w/1 -> mass dynamics through L1/2(w)
  v0/1 -> mass dynamics through L1/3(v0)
  Rgb/1 -> mass dynamics through L1/4(Rgb)
  mass dynamics through L1/5(vx_a) -> v/1, Sum/2
  mass dynamics through L1/1(p_b) -> Scope4/1, p/1
  PID Controller/1 -> mass dynamics through L1/1(U), Scope3/1
  mass dynamics through L1/3(L) -> Scope5/1
  mass dynamics through L1/6(L3b) -> L3b/1
  x3ref/1 -> Sum1/1
  mass dynamics through L1/4(x_a) -> Sum1/2

== system morus_uav_smc_DOB/hybrid multi-rotor/mass 4 model ==
  y4ref : Inport
  w : Inport  Port=2
  v0 : Inport  Port=3
  Rgb : Inport  Port=4
  PID Controller : simulink/Continuous/PID Controller  Controller=PID  TimeDomain=Continuous-time  SampleTime=-1  IntegratorMethod=Forward Euler  FilterMethod=Forward Euler  Form=Parallel  UseFilter=on  ControllerParametersSource=internal  P=kp_mv  I=ki_mv  D=kd_mv  N=100  InitialConditionSource=internal  InitialConditionForIntegrator=0  InitialConditionForFilter=0  ExternalReset=none  LimitOutput=off  UpperSaturationLimit=12  LowerSaturationLimit=-12  LinearizeAsGain=on  AntiWindupMode=clamping  Kb=1  TrackingMode=off  Kt=1  PParamMin=[]  PParamMax=[]  IParamMin=[]  IParamMax=[]  DParamMin=[]  DParamMax=[]  NParamMin=[]  NParamMax=[]  KbParamMin=[]  KbParamMax=[]  KtParamMin=[]  KtParamMax=[]  POutMin=[]  POutMax=[]  IOutMin=[]  IOutMax=[]  DOutMin=[]  DOutMax=[]  NOutMin=[]  NOutMax=[]  KbOutMin=[]  KbOutMax=[]  KtOutMin=[]  KtOutMax=[]  IntegratorOutMin=[]  IntegratorOutMax=[]  FilterOutMin=[]  FilterOutMax=[]  SumOutMin=[]  SumOutMax=[]  SumI1OutMin=[]  SumI1OutMax=[]  SumI2OutMin=[]  SumI2OutMax=[]  SumI3OutMin=[]  SumI3OutMax=[]  SumDOutMin=[]  SumDOutMax=[]  SaturationOutMin=[]  SaturationOutMax=[]  IntegratorContinuousStateAttributes=''  IntegratorStateMustResolveToSignalObject=off  IntegratorRTWStateStorageClass=Auto  FilterContinuousStateAttributes=''  FilterStateMustResolveToSignalObject=off  FilterRTWStateStorageClass=Auto  DifferentiatorICPrevScaledInput=0  DifferentiatorOutMin=[]  DifferentiatorOutMax=[]
  PID Controller1 : simulink/Continuous/PID Controller  Controller=PID  TimeDomain=Continuous-time  SampleTime=-1  IntegratorMethod=Forward Euler  FilterMethod=Forward Euler  Form=Parallel  UseFilter=on  ControllerParametersSource=internal  P=kp_mp  I=ki_mp  D=kd_mp  N=100  InitialConditionSource=internal  InitialConditionForIntegrator=0  InitialConditionForFilter=0  ExternalReset=none  LimitOutput=off  UpperSaturationLimit=12  LowerSaturationLimit=-12  LinearizeAsGain=on  AntiWindupMode=clamping  Kb=1  TrackingMode=off  Kt=1  PParamMin=[]  PParamMax=[]  IParamMin=[]  IParamMax=[]  DParamMin=[]  DParamMax=[]  NParamMin=[]  NParamMax=[]  KbParamMin=[]  KbParamMax=[]  KtParamMin=[]  KtParamMax=[]  POutMin=[]  POutMax=[]  IOutMin=[]  IOutMax=[]  DOutMin=[]  DOutMax=[]  NOutMin=[]  NOutMax=[]  KbOutMin=[]  KbOutMax=[]  KtOutMin=[]  KtOutMax=[]  IntegratorOutMin=[]  IntegratorOutMax=[]  FilterOutMin=[]  FilterOutMax=[]  SumOutMin=[]  SumOutMax=[]  SumI1OutMin=[]  SumI1OutMax=[]  SumI2OutMin=[]  SumI2OutMax=[]  SumI3OutMin=[]  SumI3OutMax=[]  SumDOutMin=[]  SumDOutMax=[]  SaturationOutMin=[]  SaturationOutMax=[]  IntegratorContinuousStateAttributes=''  IntegratorStateMustResolveToSignalObject=off  IntegratorRTWStateStorageClass=Auto  FilterContinuousStateAttributes=''  FilterStateMustResolveToSignalObject=off  FilterRTWStateStorageClass=Auto  DifferentiatorICPrevScaledInput=0  DifferentiatorOutMin=[]  DifferentiatorOutMax=[]
  Scope{1..5} (5 alike) : Scope
  Sum : Sum  Inputs=|+-
  Sum1 : Sum  Inputs=|+-
  mass dynamics through L1 : Subsystem
  p : Outport
  v : Outport  Port=2
  L4b : Outport  Port=3
  wires:
  Sum/1 -> PID Controller/1
  Sum1/1 -> PID Controller1/1
  PID Controller1/1 -> Sum/1, Scope2/1
  w/1 -> mass dynamics through L1/2(w)
  v0/1 -> mass dynamics through L1/3(v0)
  Rgb/1 -> mass dynamics through L1/4(Rgb)
  mass dynamics through L1/5(vy_a) -> Sum/2, v/1
  mass dynamics through L1/4(y_a) -> Sum1/2
  mass dynamics through L1/1(p_b) -> Scope4/1, p/1
  PID Controller/1 -> mass dynamics through L1/1(U), Scope3/1
  mass dynamics through L1/3(L) -> Scope5/1
  mass dynamics through L1/6(L4b) -> L4b/1
  y4ref/1 -> Sum1/1

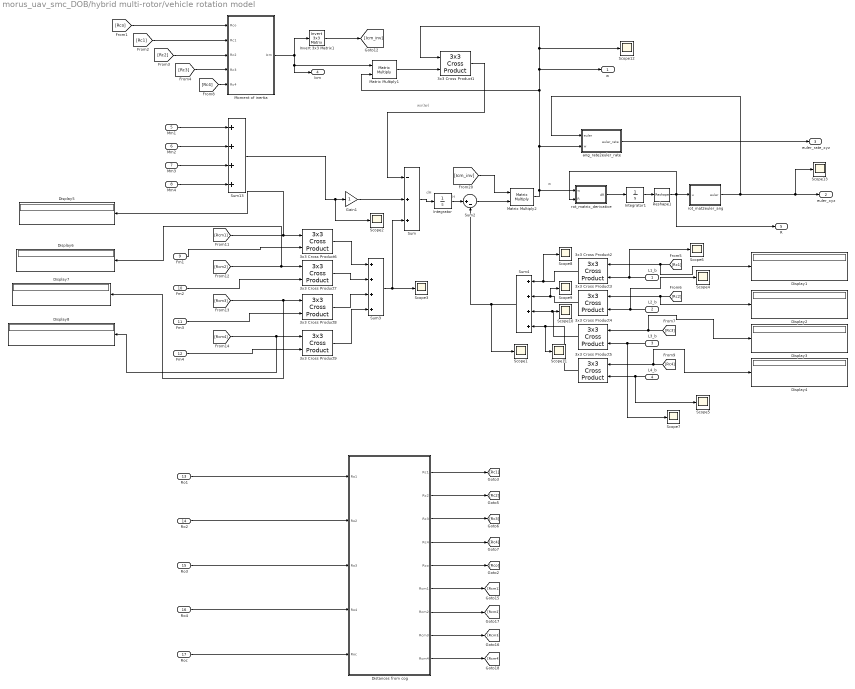
== system morus_uav_smc_DOB/hybrid multi-rotor/vehicle rotation model ==
  note: wx(Iw)
  note: w
  note: H
  note: dH
  L1_b : Inport
  L2_b : Inport  Port=2
  L3_b : Inport  Port=3
  L4_b : Inport  Port=4
  Mm1 : Inport  Port=5
  Mm2 : Inport  Port=6
  Mm3 : Inport  Port=7
  Mm4 : Inport  Port=8
  Fm1 : Inport  Port=9
  Fm2 : Inport  Port=10
  Fm3 : Inport  Port=11
  Fm4 : Inport  Port=12
  Ro1 : Inport  Port=13
  Ro2 : Inport  Port=14
  Ro3 : Inport  Port=15
  Ro4 : Inport  Port=16
  Roc : Inport  Port=17
  3x3 Cross Product{1..9} (9 alike) : aerolibutil/3x3 Cross Product
  Display{1..8} (8 alike) : Display
  Distances from cog : Subsystem
  Gain1 : Gain
  Integrator : Integrator  UpperSaturationLimit=inf* [1;1;1]  LowerSaturationLimit=-inf*[1;1;1]
  Integrator1 : Integrator  InitialCondition=eye(3)  UpperSaturationLimit=inf* [1;1;1]  LowerSaturationLimit=-inf*[1;1;1]
  Invert 3x3 Matrix1 : aerolibutil/Invert  3x3 Matrix
  Matrix Multiply1 : Product  Multiplication=Matrix(*)
  Matrix Multiply2 : Product  Multiplication=Matrix(*)
  Moment of inertia : Subsystem
  Reshape1 : Reshape  OutputDimensionality=Customize  OutputDimensions=[3,3]
  Scope{1..13} (13 alike) : Scope
  Sum : Sum  Inputs=-++
  Sum13 : Sum  Inputs=++++
  Sum2 : Sum  Inputs=|+-
  Sum3 : Sum  Inputs=++++
  Sum4 : Sum  Inputs=++++
  ang_rate2euler_rate : MATLAB Function  TreatAsAtomicUnit=on
  rot_mat2euler_ang : MATLAB Function  TreatAsAtomicUnit=on
  rot_matrix_derivative : MATLAB Function  TreatAsAtomicUnit=on
  w : Outport
  euler_xyz : Outport  Port=2
  euler_rate_xyz : Outport  Port=3
  Icm : Outport  Port=4
  R : Outport  Port=5
  wires:
  Integrator/1 -> Sum2/1
  Fm3/1 -> 3x3 Cross Product8/2
  Fm2/1 -> 3x3 Cross Product7/2
  Sum/1 -> Integrator/1
  L1_b/1 -> Scope6/1, 3x3 Cross Product2/2
  [Rc1] -> 3x3 Cross Product2/1, Display1/1
  3x3 Cross Product2/1 -> Scope8/1, Sum4/1
  3x3 Cross Product3/1 -> Scope9/1, Sum4/2
  3x3 Cross Product4/1 -> Sum4/3, Scope10/1
  3x3 Cross Product5/1 -> Scope11/1, Sum4/4
  Sum4/1 -> Scope1/1, Sum2/2
  [Rc2] -> 3x3 Cross Product3/1, Display2/1
  [Rc3] -> Display3/1, 3x3 Cross Product4/1
  [Rc4] -> Display4/1, 3x3 Cross Product5/1
  L2_b/1 -> Scope4/1, 3x3 Cross Product3/2
  L3_b/1 -> Scope7/1, 3x3 Cross Product4/2
  L4_b/1 -> Scope5/1, 3x3 Cross Product5/2
  Fm1/1 -> 3x3 Cross Product6/2
  [Rcm1] -> Display5/1, 3x3 Cross Product6/1
  Fm4/1 -> 3x3 Cross Product9/2
  [Rcm2] -> Display6/1, 3x3 Cross Product7/1
  [Rcm3] -> Display7/1, 3x3 Cross Product8/1
  [Rcm4] -> Display8/1, 3x3 Cross Product9/1
  3x3 Cross Product6/1 -> Sum3/1
  3x3 Cross Product7/1 -> Sum3/2
  3x3 Cross Product8/1 -> Sum3/3
  3x3 Cross Product9/1 -> Sum3/4
  Sum3/1 -> Sum/3, Scope3/1
  Mm1/1 -> Sum13/1
  Mm2/1 -> Sum13/2
  Mm3/1 -> Sum13/3
  Mm4/1 -> Sum13/4
  Sum13/1 -> Scope2/1, Gain1/1
  Sum2/1 -> Matrix Multiply2/2
  [Icm_inv] -> Matrix Multiply2/1
  rot_matrix_derivative/1(dR) -> Integrator1/1
  Moment of inertia/1(Icm) -> Invert 3x3 Matrix1/1, Matrix Multiply1/1, Icm/1
  [Rco] -> Moment of inertia/1(Rco)
  [Rc1] -> Moment of inertia/2(Rc1)
  [Rc2] -> Moment of inertia/3(Rc2)
  [Rc3] -> Moment of inertia/4(Rc3)
  [Rc4] -> Moment of inertia/5(Rc4)
  Ro1/1 -> Distances from cog/1(Ro1)
  Ro2/1 -> Distances from cog/2(Ro2)
  Ro3/1 -> Distances from cog/3(Ro3)
  Ro4/1 -> Distances from cog/4(Ro4)
  Roc/1 -> Distances from cog/5(Roc)
  Distances from cog/1(Rc1) -> [Rc1]
  Distances from cog/7(Rcm2) -> [Rcm2]
  Distances from cog/8(Rcm3) -> [Rcm3]
  Distances from cog/2(Rc2) -> [Rc2]
  Distances from cog/6(Rcm1) -> [Rcm1]
  Distances from cog/3(Rc3) -> [Rc3]
  Distances from cog/9(Rcm4) -> [Rcm4]
  Distances from cog/4(Rc4) -> [Rc4]
  Distances from cog/5(Rco) -> [Rco]
  Invert 3x3 Matrix1/1 -> [Icm_inv]
  Integrator1/1 -> Reshape1/1
  Reshape1/1 -> R/1, rot_mat2euler_ang/1(u), rot_matrix_derivative/2(R)
  Matrix Multiply1/1 -> 3x3 Cross Product1/2
  Matrix Multiply2/1 -> 3x3 Cross Product1/1, Scope12/1, w/1, Matrix Multiply1/2, ang_rate2euler_rate/2(w), rot_matrix_derivative/1(w)
  Gain1/1 -> Sum/2
  3x3 Cross Product1/1 -> Sum/1
  ang_rate2euler_rate/1(euler_rate) -> euler_rate_xyz/1
  rot_mat2euler_ang/1(euler) -> Scope13/1, euler_xyz/1, ang_rate2euler_rate/1(euler)

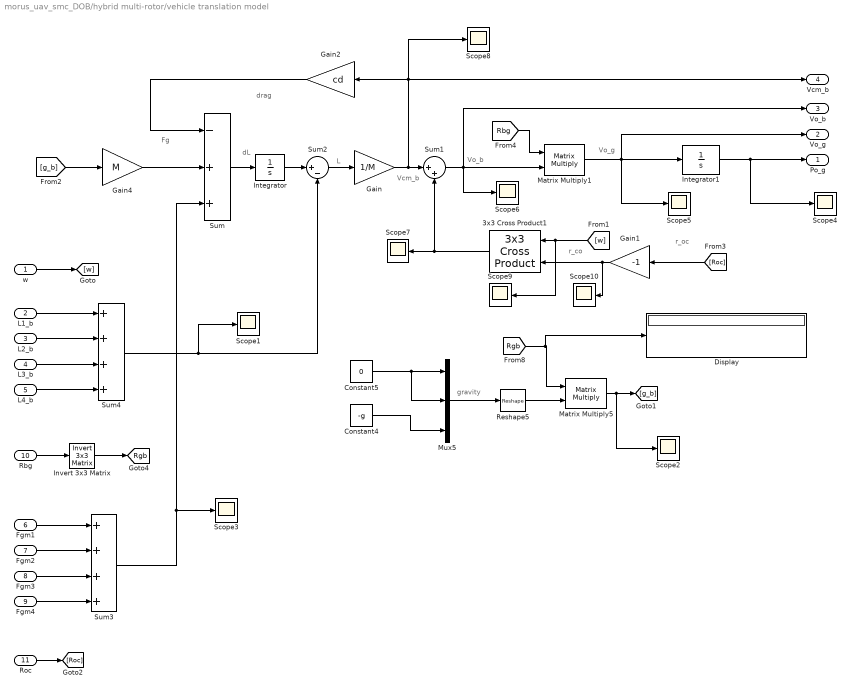
== system morus_uav_smc_DOB/hybrid multi-rotor/vehicle translation model ==
  note: Vo_g
  note: Vo_b
  note: r_oc
  note: r_co
  note: Vcm_b
  note: Fg
  note: gravity
  note: drag
  note: dL
  note: L
  w : Inport
  L1_b : Inport  Port=2
  L2_b : Inport  Port=3
  L3_b : Inport  Port=4
  L4_b : Inport  Port=5
  Fgm1 : Inport  Port=6
  Fgm2 : Inport  Port=7
  Fgm3 : Inport  Port=8
  Fgm4 : Inport  Port=9
  Rbg : Inport  Port=10
  Roc : Inport  Port=11
  3x3 Cross Product1 : aerolibutil/3x3 Cross Product
  Constant4 : Constant  Value=-g
  Constant5 : Constant  Value=0
  Display : Display
  Gain : Gain  Gain=1/M
  Gain1 : Gain  Gain=-1
  Gain2 : Gain  Gain=cd
  Gain4 : Gain  Gain=M
  Integrator : Integrator  UpperSaturationLimit=inf* [1;1;1]  LowerSaturationLimit=-inf*[1;1;1]
  Integrator1 : Integrator  InitialCondition=[-0.5;0.5;0.2]  UpperSaturationLimit=[inf,inf,inf]  LowerSaturationLimit=[-inf,-inf,-inf]
  Invert 3x3 Matrix : aerolibutil/Invert  3x3 Matrix
  Matrix Multiply1 : Product  Multiplication=Matrix(*)
  Matrix Multiply5 : Product  Multiplication=Matrix(*)
  Mux5 : Mux  Inputs=3
  Reshape5 : Reshape  OutputDimensionality=Customize  OutputDimensions=[3,1]
  Scope{1..10} (10 alike) : Scope
  Sum : Sum  Inputs=-++
  Sum1 : Sum  Inputs=|++
  Sum2 : Sum  Inputs=|+-
  Sum3 : Sum  Inputs=++++
  Sum4 : Sum  Inputs=++++
  Po_g : Outport
  Vo_g : Outport  Port=2
  Vo_b : Outport  Port=3
  Vcm_b : Outport  Port=4
  tag scope: Rgb=global
  wires:
  Gain4/1 -> Sum/2
  Gain2/1 -> Sum/1
  [g_b] -> Gain4/1
  [w] -> Scope9/1, 3x3 Cross Product1/1
  Reshape5/1 -> Matrix Multiply5/2
  [Rgb] -> Display/1, Matrix Multiply5/1
  Mux5/1 -> Reshape5/1
  Constant4/1 -> Mux5/3
  Constant5/1 -> Mux5/1, Mux5/2
  Sum/1 -> Integrator/1
  w/1 -> [w]
  L1_b/1 -> Sum4/1
  L2_b/1 -> Sum4/2
  L3_b/1 -> Sum4/3
  L4_b/1 -> Sum4/4
  Matrix Multiply5/1 -> Scope2/1, [g_b]
  Fgm1/1 -> Sum3/1
  Fgm2/1 -> Sum3/2
  Fgm3/1 -> Sum3/3
  Fgm4/1 -> Sum3/4
  Sum4/1 -> Sum2/2, Scope1/1
  Sum3/1 -> Sum/3, Scope3/1
  Roc/1 -> [Roc]
  [Roc] -> Gain1/1
  Gain1/1 -> Scope10/1, 3x3 Cross Product1/2
  Gain/1 -> Scope8/1, Vcm_b/1, Gain2/1, Sum1/1
  Sum1/1 -> Scope6/1, Matrix Multiply1/2, Vo_b/1
  Rbg/1 -> Invert 3x3 Matrix/1
  Invert 3x3 Matrix/1 -> [Rgb]
  [Rbg] -> Matrix Multiply1/1
  Matrix Multiply1/1 -> Scope5/1, Vo_g/1, Integrator1/1
  Integrator1/1 -> Scope4/1, Po_g/1
  3x3 Cross Product1/1 -> Scope7/1, Sum1/2
  Integrator/1 -> Sum2/1
  Sum2/1 -> Gain/1

== system morus_uav_smc_DOB/attitude control/pitch control/Subsystem ==
  note: q_ref''
  pitch_ref : Inport
  Gain1 : Gain  Gain=1/(Tf1*Tf2)
  Gain2 : Gain  Gain=Tf1+Tf2
  Integrator1 : Integrator
  Integrator2 : Integrator
  Sum1 : Sum  Inputs=|+--
  q_ref : Outport
  q_ref' : Outport  Port=2
  q_ref'' : Outport  Port=3
  wires:
  Gain1/1 -> q_ref''/1, Integrator1/1
  Integrator1/1 -> q_ref'/1, Gain2/1, Integrator2/1
  Sum1/1 -> Gain1/1
  pitch_ref/1 -> Sum1/1
  Integrator2/1 -> q_ref/1, Sum1/2
  Gain2/1 -> Sum1/3

== system morus_uav_smc_DOB/attitude control/pitch control/Subsystem1 ==
  note: 0.06
  note: 1
  note: 35
  note: s
  e : Inport
  q_ref' : Inport  Port=2
  q_ref'' : Inport  Port=3
  pitch_r : Inport  Port=4
  Dead Zone : DeadZone  LowerValue=-0.00001  UpperValue=0.00001  SaturateOnIntegerOverflow=on
  Gain : Gain  Gain=0
  Gain2 : Gain  Gain=5
  Gain7 : Gain  Gain=13
  Integrator : Integrator
  Sum : Sum  Inputs=+++
  Sum1 : Sum  Inputs=+++
  Sum3 : Sum  Inputs=|+-
  Trigonometric Function : Trigonometry  Operator=tanh
  "lambda " : Gain  Gain=0
  u_r : Outport
  wires:
  Sum/1 -> Dead Zone/1
  "lambda "/1 -> Sum/2
  Gain2/1 -> Sum1/1
  Integrator/1 -> Gain/1
  pitch_r/1 -> Sum3/2
  q_ref'/1 -> Sum3/1
  Trigonometric Function/1 -> Gain7/1
  Gain/1 -> Sum/1
  Sum1/1 -> u_r/1  "u_r"
  Gain7/1 -> Sum1/2
  e/1 -> "lambda "/1, Integrator/1, Gain2/1
  Dead Zone/1 -> Trigonometric Function/1
  Sum3/1 -> Sum/3
  q_ref''/1 -> Sum1/3

== system morus_uav_smc_DOB/attitude control/roll control/Subsystem ==
  note: q_ref''
  roll_ref : Inport
  Gain1 : Gain  Gain=1/(Tf1*Tf2)
  Gain2 : Gain  Gain=Tf1+Tf2
  Integrator1 : Integrator
  Integrator2 : Integrator
  Sum1 : Sum  Inputs=|+--
  q_ref : Outport
  q_ref' : Outport  Port=2
  q_ref'' : Outport  Port=3
  wires:
  Gain1/1 -> q_ref''/1, Integrator1/1
  Integrator1/1 -> q_ref'/1, Gain2/1, Integrator2/1
  Sum1/1 -> Gain1/1
  roll_ref/1 -> Sum1/1
  Integrator2/1 -> q_ref/1, Sum1/2
  Gain2/1 -> Sum1/3

== system morus_uav_smc_DOB/attitude control/roll control/Subsystem1 ==
  note: s
  In1 : Inport
  In2 : Inport  Port=2
  roll_r : Inport  Port=3
  In4 : Inport  Port=4
  Dead Zone : DeadZone  LowerValue=-0.00001  UpperValue=0.00001  SaturateOnIntegerOverflow=on
  Gain : Gain  Gain=0
  Gain2 : Gain  Gain=5
  Gain7 : Gain  Gain=13
  Integrator : Integrator
  Sum : Sum  Inputs=+-|
  Sum1 : Sum  Inputs=+++
  Sum3 : Sum  Inputs=+++
  Trigonometric Function : Trigonometry  Operator=tanh
  "lambda " : Gain  Gain=0
  Out1 : Outport
  wires:
  Gain7/1 -> Sum3/2
  In2/1 -> Sum/1
  Dead Zone/1 -> Trigonometric Function/1
  In4/1 -> Sum3/3
  Sum3/1 -> Out1/1
  In1/1 -> Gain2/1, Integrator/1, "lambda "/1
  Trigonometric Function/1 -> Gain7/1
  Sum/1 -> Sum1/3
  Sum1/1 -> Dead Zone/1
  Gain2/1 -> Sum3/1
  "lambda "/1 -> Sum1/2
  roll_r/1 -> Sum/2
  Integrator/1 -> Gain/1
  Gain/1 -> Sum1/1

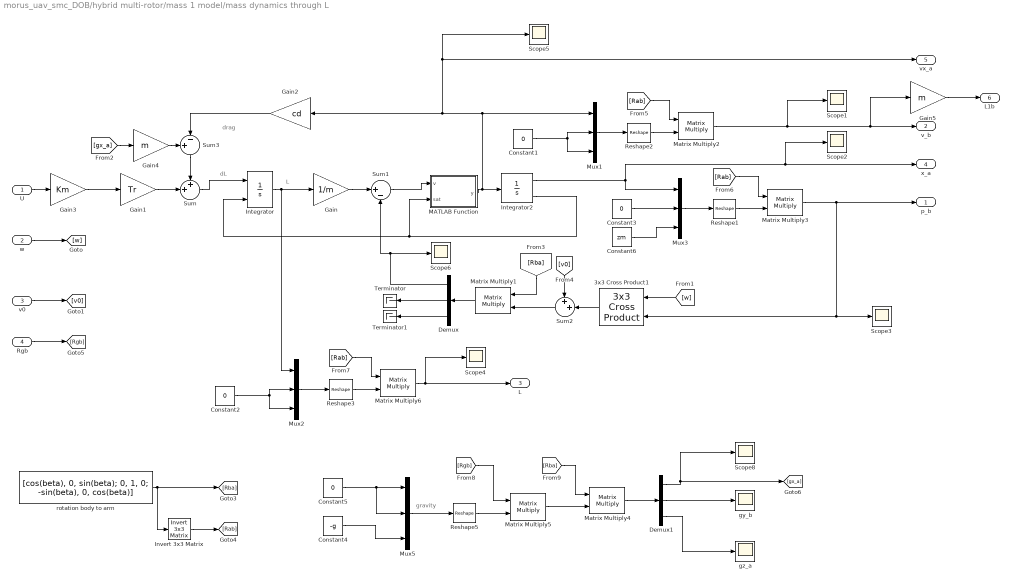
== system morus_uav_smc_DOB/hybrid multi-rotor/mass 1 model/mass dynamics through L ==
  note: L
  note: dL
  note: drag
  note: gravity
  U : Inport
  w : Inport  Port=2
  v0 : Inport  Port=3
  Rgb : Inport  Port=4
  3x3 Cross Product1 : aerolibutil/3x3 Cross Product
  Constant{1..3,5} (4 alike) : Constant  Value=0
  Constant4 : Constant  Value=-g
  Constant6 : Constant  Value=zm
  Demux : Demux  Outputs=3
  Demux1 : Demux  Outputs=3
  Gain : Gain  Gain=1/m
  Gain1 : Gain  Gain=Tr
  Gain2 : Gain  Gain=cd
  Gain3 : Gain  Gain=Km
  Gain4 : Gain  Gain=m
  Gain5 : Gain  Gain=m
  Integrator : Integrator  ExternalReset=level  UpperSaturationLimit=m*12  LowerSaturationLimit=-m*12
  Integrator2 : Integrator  InitialCondition=lm/2  LimitOutput=on  UpperSaturationLimit=lm+0.01  LowerSaturationLimit=-0.01  ShowSaturationPort=on
  Invert 3x3 Matrix : aerolibutil/Invert  3x3 Matrix
  MATLAB Function : MATLAB Function  TreatAsAtomicUnit=on
  Matrix Multiply{1..6} (6 alike) : Product  Multiplication=Matrix(*)
  Mux{1..3,5} (4 alike) : Mux  Inputs=3
  Reshape{1..3,5} (4 alike) : Reshape  OutputDimensionality=Customize  OutputDimensions=[3,1]
  Scope{1..6,8} (7 alike) : Scope
  Sum : Sum  Inputs=++|
  Sum1 : Sum  Inputs=|+-
  Sum2 : Sum  Inputs=++|
  Sum3 : Sum  Inputs=+-|
  Terminator : Terminator
  Terminator1 : Terminator
  gy_b : Scope
  gz_a : Scope
  rotation body to arm : Constant  Value=[cos(beta), 0, sin(beta); 0, 1, 0; -sin(beta), 0, cos(beta)]
  p_b : Outport
  v_b : Outport  Port=2
  L : Outport  Port=3
  x_a : Outport  Port=4
  vx_a : Outport  Port=5
  L1b : Outport  Port=6
  wires:
  w/1 -> [w]
  Sum/1 -> Integrator/1
  U/1 -> Gain3/1
  Gain3/1 -> Gain1/1
  v0/1 -> [v0]
  Rgb/1 -> [Rgb]
  rotation body to arm/1 -> [Rba], Invert 3x3 Matrix/1
  Invert 3x3 Matrix/1 -> [Rab]
  Constant5/1 -> Mux5/2, Mux5/1
  Constant4/1 -> Mux5/3
  [Rba] -> Matrix Multiply4/1
  Matrix Multiply4/1 -> Demux1/1
  Mux5/1 -> Reshape5/1
  [Rgb] -> Matrix Multiply5/1
  Matrix Multiply5/1 -> Matrix Multiply4/2
  Reshape5/1 -> Matrix Multiply5/2
  Demux1/1 -> Scope8/1, [gx_a]
  Demux1/2 -> gy_b/1
  Demux1/3 -> gz_a/1
  [w] -> 3x3 Cross Product1/1
  Mux3/1 -> Reshape1/1
  3x3 Cross Product1/1 -> Sum2/2
  [v0] -> Sum2/1
  Sum2/1 -> Matrix Multiply1/2
  [Rba] -> Matrix Multiply1/1
  Integrator2/1 -> Mux3/1, Scope2/1, x_a/1
  Constant3/1 -> Mux3/2
  Gain/1 -> Sum1/1
  Mux1/1 -> Reshape2/1
  Constant1/1 -> Mux1/2, Mux1/3
  Reshape2/1 -> Matrix Multiply2/2
  [Rab] -> Matrix Multiply2/1
  [Rab] -> Matrix Multiply3/1
  Reshape1/1 -> Matrix Multiply3/2
  Matrix Multiply2/1 -> Scope1/1, Gain5/1, v_b/1
  Matrix Multiply3/1 -> Scope3/1, 3x3 Cross Product1/2, p_b/1
  Matrix Multiply1/1 -> Demux/1
  Demux/2 -> Terminator/1
  Demux/3 -> Terminator1/1
  Gain2/1 -> Sum3/2
  [gx_a] -> Gain4/1
  Sum3/1 -> Sum/1
  Gain1/1 -> Sum/2
  Gain4/1 -> Sum3/1
  Integrator2/2 -> MATLAB Function/2(sat), Integrator/2
  Sum1/1 -> MATLAB Function/1(v)
  Mux2/1 -> Reshape3/1
  Constant2/1 -> Mux2/2, Mux2/3
  Reshape3/1 -> Matrix Multiply6/2
  [Rab] -> Matrix Multiply6/1
  Matrix Multiply6/1 -> Scope4/1, L/1
  Integrator/1 -> Mux2/1, Gain/1
  Demux/1 -> Sum1/2, Scope6/1
  MATLAB Function/1(y) -> Integrator2/1, Gain2/1, Scope5/1, vx_a/1, Mux1/1
  Constant6/1 -> Mux3/3
  Gain5/1 -> L1b/1
